simulink model "admittance_control_fra"  (R2023a)
settings: Solver=VariableStepAuto  StartTime=0.0  StopTime=tf  RelTol=1e-3
undefined symbols (not defined in the file): dqi, K, KD, KDt, KP, KPt, Mt, qi, robot, xr
settings Model: Creator=franc  LastModifiedBy=franc

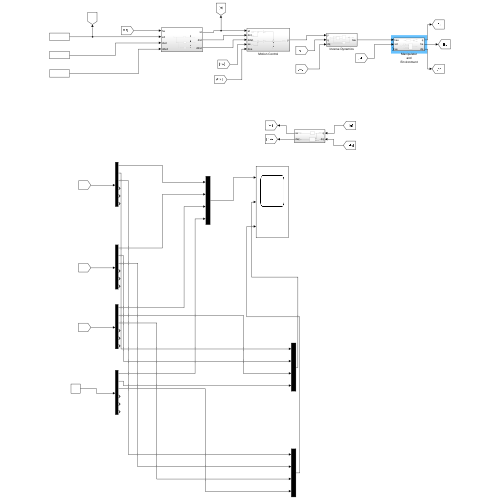
[thumbnail: Simulink's stored preview of the top-level diagram]
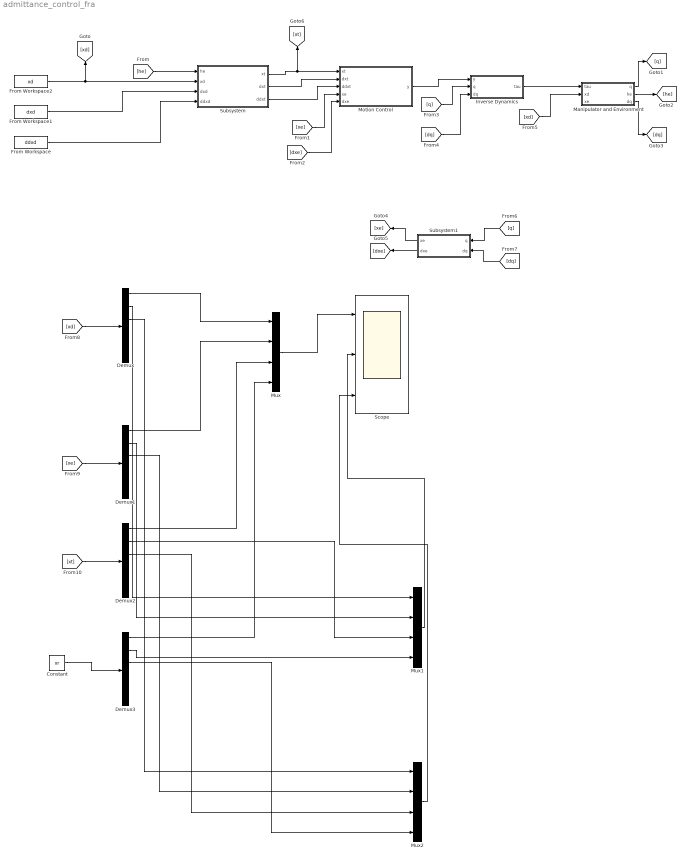
== system admittance_control_fra ==
  Constant : Constant  Value=xr
  Demux{,1..3} (4 alike) : Demux  Outputs=6
  From Workspace : FromWorkspace  VariableName=ddxd
  From Workspace1 : FromWorkspace  VariableName=dxd
  From Workspace2 : FromWorkspace  VariableName=xd
  Inverse Dynamics : Subsystem
  Manipulator and Environment : Subsystem
  Motion Control : Subsystem
  Mux : Mux
  Mux1 : Mux
  Mux2 : Mux
  Scope : Scope  NumInputPorts=3
  Subsystem : Subsystem
  Subsystem1 : Subsystem
  wires:
  From Workspace2/1 -> [xd], Subsystem/2(xd)
  From Workspace1/1 -> Subsystem/3(dxd)
  From Workspace/1 -> Subsystem/4(ddxd)
  [he] -> Subsystem/1(he)
  Subsystem/1(xt) -> Motion Control/1(xt), [xt]
  Subsystem/2(dxt) -> Motion Control/2(dxt)
  Subsystem/3(ddxt) -> Motion Control/3(ddxt)
  [xe] -> Motion Control/4(xe)
  [dxe] -> Motion Control/5(dxe)
  Motion Control/1(y) -> Inverse Dynamics/1(y)
  [q] -> Inverse Dynamics/2(q)
  [dq] -> Inverse Dynamics/3(dq)
  Inverse Dynamics/1(tau) -> Manipulator and Environment/1(tau)
  [xd] -> Manipulator and Environment/2(xd)
  Manipulator and Environment/1(q) -> [q]
  Manipulator and Environment/2(he) -> [he]
  Manipulator and Environment/3(dq) -> [dq]
  Subsystem1/1(xe) -> [xe]
  Subsystem1/2(dxe) -> [dxe]
  [q] -> Subsystem1/1(q)
  [dq] -> Subsystem1/2(dq)
  Constant/1 -> Demux3/1
  [xt] -> Demux2/1
  [xe] -> Demux1/1
  [xd] -> Demux/1
  Demux/1 -> Mux/1
  Demux1/1 -> Mux/2
  Demux2/1 -> Mux/3
  Demux3/1 -> Mux/4
  Mux/1 -> Scope/1
  Mux1/1 -> Scope/2
  Mux2/1 -> Scope/3
  Demux3/3 -> Mux2/4
  Demux2/3 -> Mux2/3
  Demux1/3 -> Mux2/2
  Demux/3 -> Mux2/1
  Demux3/2 -> Mux1/4
  Demux2/2 -> Mux1/3
  Demux1/2 -> Mux1/2
  Demux/2 -> Mux1/1

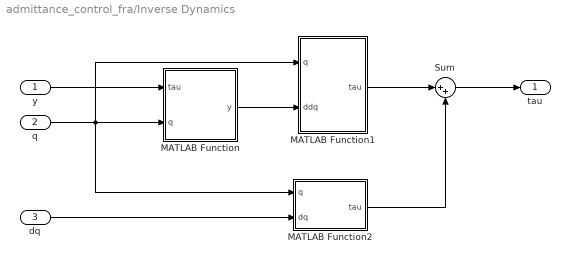
== system admittance_control_fra/Inverse Dynamics ==
  y : Inport
  q : Inport  Port=2
  dq : Inport  Port=3
  MATLAB Function : MATLAB Function  TreatAsAtomicUnit=on
  MATLAB Function1 : MATLAB Function  TreatAsAtomicUnit=on
  MATLAB Function2 : MATLAB Function  TreatAsAtomicUnit=on
  Sum : Sum  Inputs=|++
  tau : Outport
  wires:
  y/1 -> MATLAB Function/1(tau)
  q/1 -> MATLAB Function/2(q), MATLAB Function2/1(q), MATLAB Function1/1(q)
  MATLAB Function/1(y) -> MATLAB Function1/2(ddq)
  dq/1 -> MATLAB Function2/2(dq)
  MATLAB Function1/1(tau) -> Sum/1
  MATLAB Function2/1(tau) -> Sum/2
  Sum/1 -> tau/1

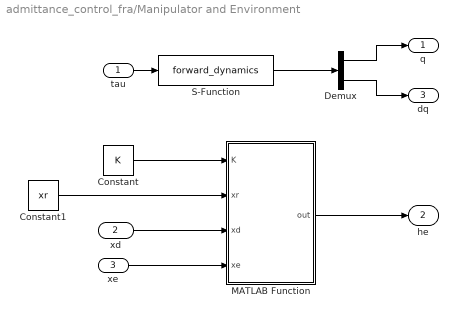
== system admittance_control_fra/Manipulator and Environment ==
  tau : Inport
  xd : Inport  Port=2
  xe : Inport  Port=3
  Constant : Constant  Value=K
  Constant1 : Constant  Value=xr
  Demux : Demux  Outputs=2
  MATLAB Function : MATLAB Function  TreatAsAtomicUnit=on
  S-Function : S-Function  FunctionName=forward_dynamics  Parameters=robot,qi,dqi  SFunctionDeploymentMode=off  EnableBusSupport=off
  q : Outport
  he : Outport  Port=2
  dq : Outport  Port=3
  wires:
  tau/1 -> S-Function/1
  xd/1 -> MATLAB Function/3(xd)
  Constant/1 -> MATLAB Function/1(K)
  Constant1/1 -> MATLAB Function/2(xr)
  MATLAB Function/1(out) -> he/1
  S-Function/1 -> Demux/1
  Demux/1 -> q/1
  Demux/2 -> dq/1
  xe/1 -> MATLAB Function/4(xe)

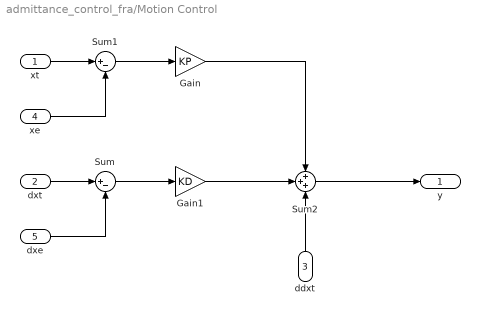
== system admittance_control_fra/Motion Control ==
  xt : Inport
  dxt : Inport  Port=2
  ddxt : Inport  Port=3
  xe : Inport  Port=4
  dxe : Inport  Port=5
  Gain : Gain  Gain=KP
  Gain1 : Gain  Gain=KD
  Sum : Sum  Inputs=|+-
  Sum1 : Sum  Inputs=|+-
  Sum2 : Sum  Inputs=+++
  y : Outport
  wires:
  dxt/1 -> Sum/1
  dxe/1 -> Sum/2
  xe/1 -> Sum1/2
  xt/1 -> Sum1/1
  Sum/1 -> Gain1/1
  Sum1/1 -> Gain/1
  Sum2/1 -> y/1
  Gain/1 -> Sum2/1
  Gain1/1 -> Sum2/2
  ddxt/1 -> Sum2/3

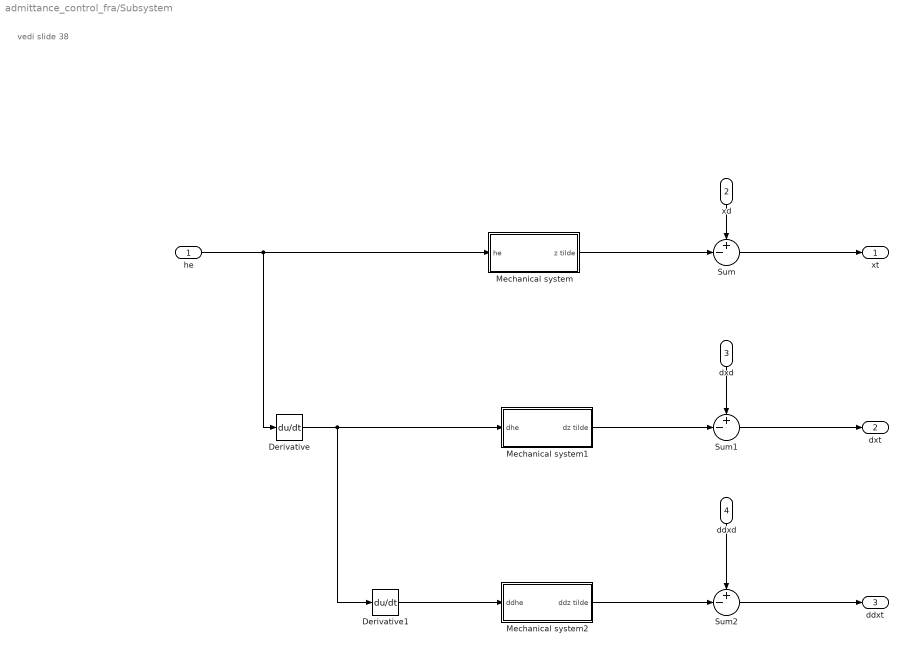
== system admittance_control_fra/Subsystem ==
  note: vedi slide 38
  he : Inport
  xd : Inport  Port=2
  dxd : Inport  Port=3
  ddxd : Inport  Port=4
  Derivative : Derivative
  Derivative1 : Derivative
  Mechanical system : Subsystem
  Mechanical system1 : Subsystem
  Mechanical system2 : Subsystem
  Sum : Sum  Inputs=+-|
  Sum1 : Sum  Inputs=+-|
  Sum2 : Sum  Inputs=+-|
  xt : Outport
  dxt : Outport  Port=2
  ddxt : Outport  Port=3
  wires:
  xd/1 -> Sum/1
  he/1 -> Mechanical system/1(he), Derivative/1
  dxd/1 -> Sum1/1
  Sum1/1 -> dxt/1
  ddxd/1 -> Sum2/1
  Sum2/1 -> ddxt/1
  Derivative/1 -> Mechanical system1/1(dhe), Derivative1/1
  Mechanical system/1(z tilde) -> Sum/2
  Mechanical system1/1(dz tilde) -> Sum1/2
  Derivative1/1 -> Mechanical system2/1(ddhe)
  Mechanical system2/1(ddz tilde) -> Sum2/2
  Sum/1 -> xt/1

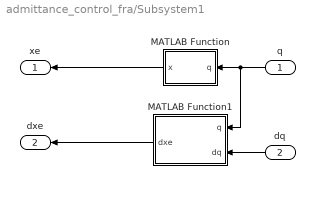
== system admittance_control_fra/Subsystem1 ==
  q : Inport
  dq : Inport  Port=2
  MATLAB Function : MATLAB Function  TreatAsAtomicUnit=on
  MATLAB Function1 : MATLAB Function  TreatAsAtomicUnit=on
  xe : Outport
  dxe : Outport  Port=2
  wires:
  q/1 -> MATLAB Function1/1(q), MATLAB Function/1(q)
  dq/1 -> MATLAB Function1/2(dq)
  MATLAB Function/1(x) -> xe/1
  MATLAB Function1/1(dxe) -> dxe/1

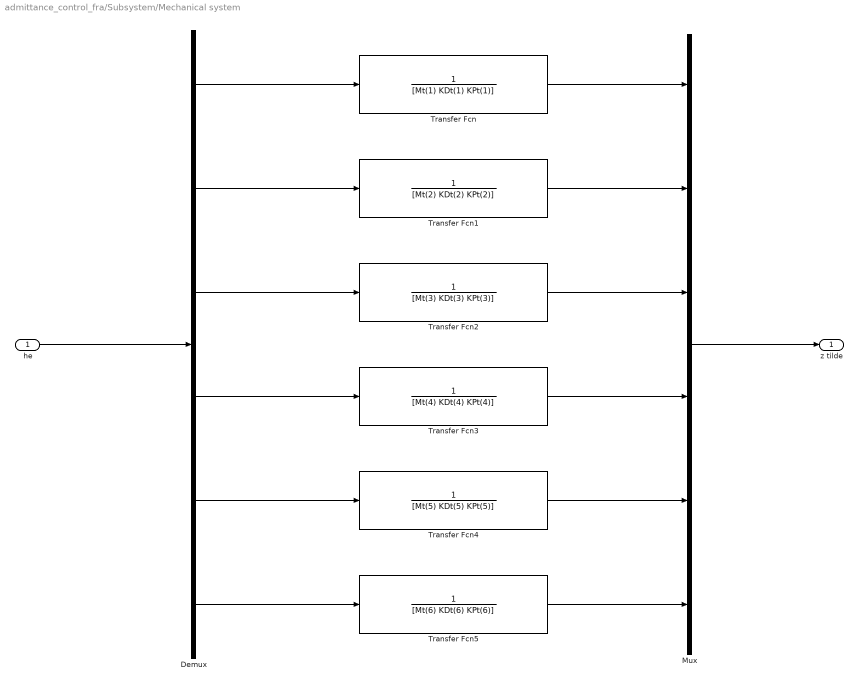
== system admittance_control_fra/Subsystem/Mechanical system ==
  he : Inport
  Demux : Demux  Outputs=6
  Mux : Mux  Inputs=6
  Transfer Fcn : TransferFcn  Denominator=[Mt(1) KDt(1) KPt(1)]
  Transfer Fcn1 : TransferFcn  Denominator=[Mt(2) KDt(2) KPt(2)]
  Transfer Fcn2 : TransferFcn  Denominator=[Mt(3) KDt(3) KPt(3)]
  Transfer Fcn3 : TransferFcn  Denominator=[Mt(4) KDt(4) KPt(4)]
  Transfer Fcn4 : TransferFcn  Denominator=[Mt(5) KDt(5) KPt(5)]
  Transfer Fcn5 : TransferFcn  Denominator=[Mt(6) KDt(6) KPt(6)]
  z tilde : Outport
  wires:
  he/1 -> Demux/1
  Demux/1 -> Transfer Fcn/1
  Demux/3 -> Transfer Fcn2/1
  Demux/2 -> Transfer Fcn1/1
  Demux/4 -> Transfer Fcn3/1
  Demux/5 -> Transfer Fcn4/1
  Demux/6 -> Transfer Fcn5/1
  Transfer Fcn/1 -> Mux/1
  Transfer Fcn1/1 -> Mux/2
  Transfer Fcn2/1 -> Mux/3
  Transfer Fcn3/1 -> Mux/4
  Transfer Fcn5/1 -> Mux/6
  Transfer Fcn4/1 -> Mux/5
  Mux/1 -> z tilde/1

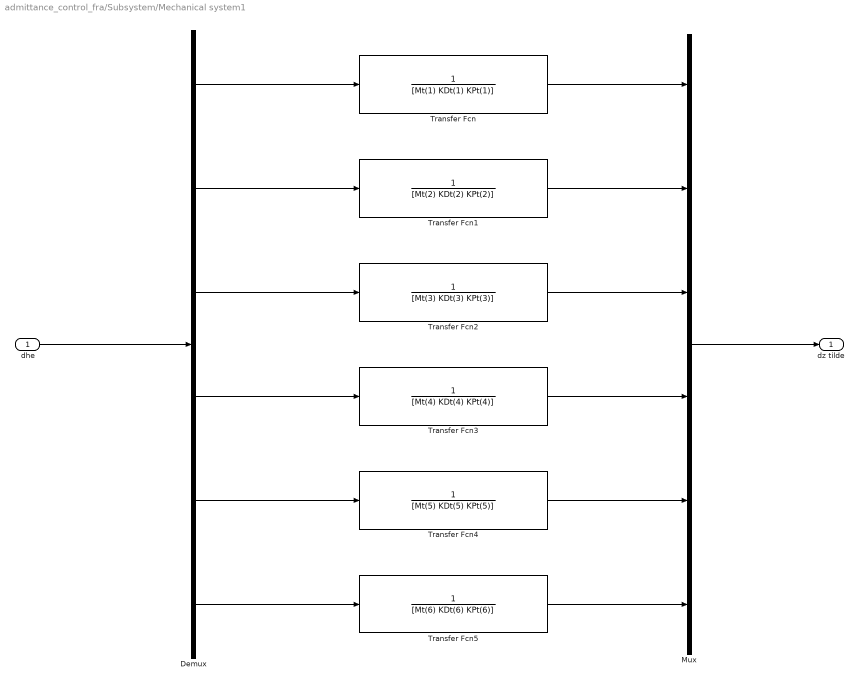
== system admittance_control_fra/Subsystem/Mechanical system1 ==
  dhe : Inport
  Demux : Demux  Outputs=6
  Mux : Mux  Inputs=6
  Transfer Fcn : TransferFcn  Denominator=[Mt(1) KDt(1) KPt(1)]
  Transfer Fcn1 : TransferFcn  Denominator=[Mt(2) KDt(2) KPt(2)]
  Transfer Fcn2 : TransferFcn  Denominator=[Mt(3) KDt(3) KPt(3)]
  Transfer Fcn3 : TransferFcn  Denominator=[Mt(4) KDt(4) KPt(4)]
  Transfer Fcn4 : TransferFcn  Denominator=[Mt(5) KDt(5) KPt(5)]
  Transfer Fcn5 : TransferFcn  Denominator=[Mt(6) KDt(6) KPt(6)]
  dz tilde : Outport
  wires:
  dhe/1 -> Demux/1
  Demux/1 -> Transfer Fcn/1
  Demux/3 -> Transfer Fcn2/1
  Demux/2 -> Transfer Fcn1/1
  Demux/4 -> Transfer Fcn3/1
  Demux/5 -> Transfer Fcn4/1
  Demux/6 -> Transfer Fcn5/1
  Transfer Fcn/1 -> Mux/1
  Transfer Fcn1/1 -> Mux/2
  Transfer Fcn2/1 -> Mux/3
  Transfer Fcn3/1 -> Mux/4
  Transfer Fcn5/1 -> Mux/6
  Transfer Fcn4/1 -> Mux/5
  Mux/1 -> dz tilde/1

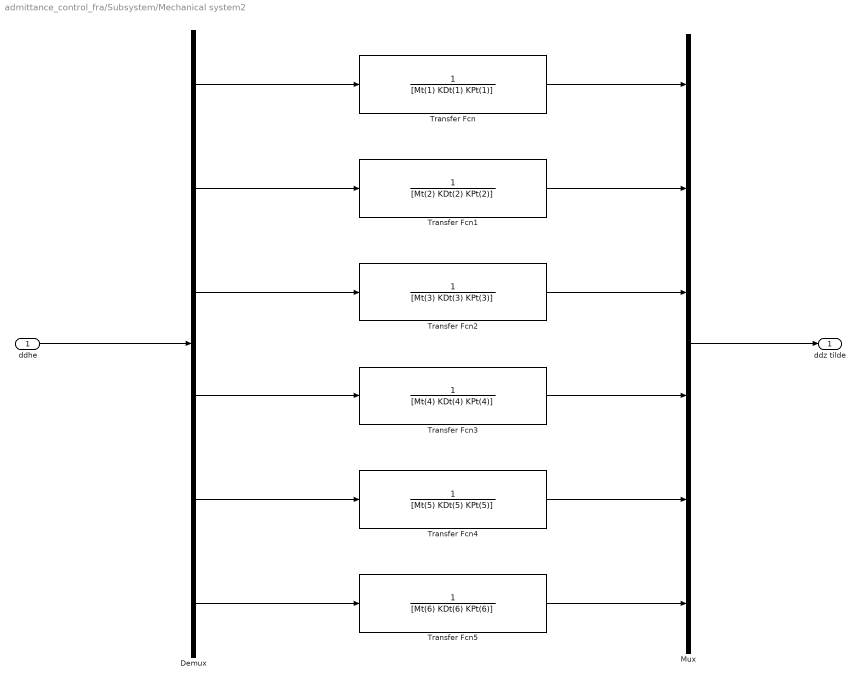
== system admittance_control_fra/Subsystem/Mechanical system2 ==
  ddhe : Inport
  Demux : Demux  Outputs=6
  Mux : Mux  Inputs=6
  Transfer Fcn : TransferFcn  Denominator=[Mt(1) KDt(1) KPt(1)]
  Transfer Fcn1 : TransferFcn  Denominator=[Mt(2) KDt(2) KPt(2)]
  Transfer Fcn2 : TransferFcn  Denominator=[Mt(3) KDt(3) KPt(3)]
  Transfer Fcn3 : TransferFcn  Denominator=[Mt(4) KDt(4) KPt(4)]
  Transfer Fcn4 : TransferFcn  Denominator=[Mt(5) KDt(5) KPt(5)]
  Transfer Fcn5 : TransferFcn  Denominator=[Mt(6) KDt(6) KPt(6)]
  ddz tilde : Outport
  wires:
  ddhe/1 -> Demux/1
  Demux/1 -> Transfer Fcn/1
  Demux/3 -> Transfer Fcn2/1
  Demux/2 -> Transfer Fcn1/1
  Demux/4 -> Transfer Fcn3/1
  Demux/5 -> Transfer Fcn4/1
  Demux/6 -> Transfer Fcn5/1
  Transfer Fcn/1 -> Mux/1
  Transfer Fcn1/1 -> Mux/2
  Transfer Fcn2/1 -> Mux/3
  Transfer Fcn3/1 -> Mux/4
  Transfer Fcn5/1 -> Mux/6
  Transfer Fcn4/1 -> Mux/5
  Mux/1 -> ddz tilde/1

== matlab function admittance_control_fra/Inverse Dynamics/MATLAB Function1 ==
  data: q input; tau output; ddq input
function tau = B(q,ddq)
tau = zeros(3,1);
tau = get_B_as_7(q(1),q(3)) * ddq;

== matlab function admittance_control_fra/Inverse Dynamics/MATLAB Function ==
  data: tau input; y output; q input
function y = JA_inv(tau,q)
y = zeros(3,1);
y = get_Ja_inverse_as_9(q(1),q(2),q(3)) * tau;

== matlab function admittance_control_fra/Inverse Dynamics/MATLAB Function2 ==
  data: q input; tau output; dq input
function tau = n(q,dq)
tau = zeros(3,1);
tau = get_n_as_7(q(1),q(3),dq(1),dq(3));

== matlab function admittance_control_fra/Manipulator and Environment/MATLAB Function ==
  data: K input; xr input; xd input; out output; xe input
function out = hde(K, xr, xd, xe)
%consider the interaction only in z direction
% if the end effector touch the environment 
he = zeros(6,1);

if xe(3) > xr(3)
    %The interaction force between the end-effector and the environment is
    dxrd = xd-xr;
    dxed = xd-xe;
    dxre = dxrd-dxed;
    he = K*dxre;
end

out = he;

== matlab function admittance_control_fra/Subsystem1/MATLAB Function ==
  data: q input; x output
function x = K(q)

x = get_k_as_9(q(1),q(2),q(3));

== matlab function admittance_control_fra/Subsystem1/MATLAB Function1 ==
  data: q input; dxe output; dq input
function dxe = velocity_K(q,dq)
dxe = zeros(6,1);
dxe = get_Ja_as_9(q(1),q(2),q(3))*dq;
